simulink model "Task1_Direct_MRAC"  (R2024b)
settings: Solver=ode45  StartTime=0.0  StopTime=60  MaxStep=0.01  RelTol=1e-7  AbsTol=1e-9
Description:
  | Task 1 direct MRAC. The plant, reference model, command, controller, regressor, and adaptive laws are contained in the MATLAB Function block.
  | Set Command Case to 1 for the step command or 2 for the five-tone PE command.
  | Results are shown only in Scope and Display blocks.
settings Model: Creator=LAPTOPASADI  LastModifiedBy=LAPTOPASADI
settings DataIOCC: SaveOutput=off  SignalLogging=off  SaveTime=off  ReturnWorkspaceOutputs=off

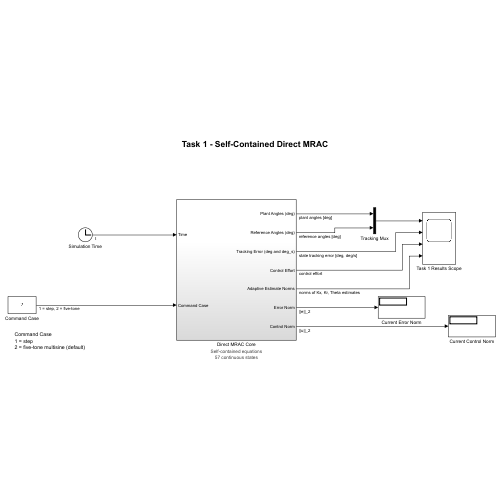
[thumbnail: Simulink's stored preview of the top-level diagram]
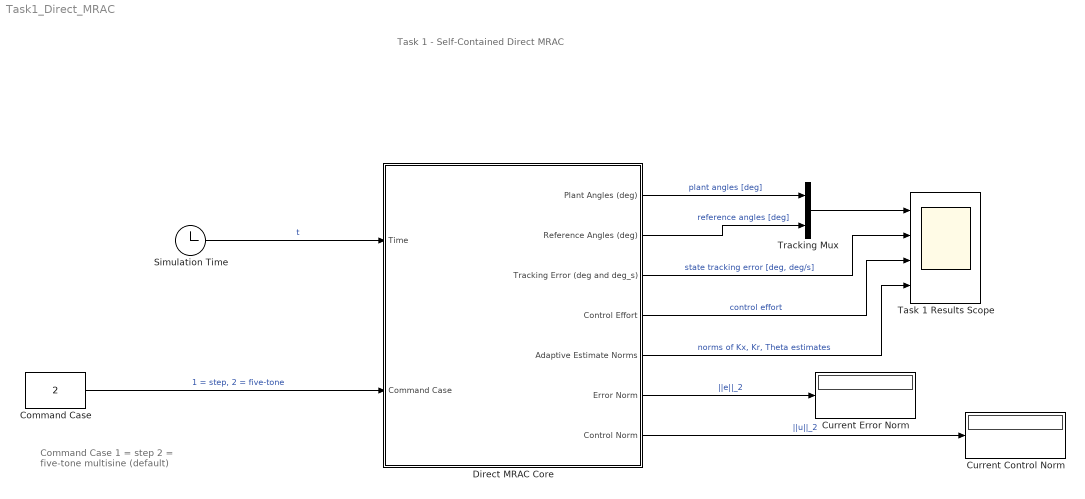
== system Task1_Direct_MRAC ==
  note: Task 1 - Self-Contained Direct MRAC
  note: Command Case
      | 1 = step
      | 2 = five-tone multisine (default)
  Command Case : Constant  Value=2  OutDataTypeStr=double
  Current Control Norm : Display
  Current Error Norm : Display
  Direct MRAC Core : Subsystem
      settings: AttributesFormatString=Self-contained equations\n57 continuous states
  Simulation Time : Clock
  Task 1 Results Scope : Scope  NumInputPorts=4
  Tracking Mux : Mux  Inputs=2
  wires:
  Simulation Time/1 -> Direct MRAC Core/1(Time)  "t"
  Command Case/1 -> Direct MRAC Core/2(Command Case)  "1 = step, 2 = five-tone"
  Direct MRAC Core/1(Plant Angles (deg)) -> Tracking Mux/1  "plant angles [deg]"
  Direct MRAC Core/2(Reference Angles (deg)) -> Tracking Mux/2  "reference angles [deg]"
  Tracking Mux/1 -> Task 1 Results Scope/1
  Direct MRAC Core/3(Tracking Error (deg and deg_s)) -> Task 1 Results Scope/2  "state tracking error [deg, deg/s]"
  Direct MRAC Core/4(Control Effort) -> Task 1 Results Scope/3  "control effort"
  Direct MRAC Core/5(Adaptive Estimate Norms) -> Task 1 Results Scope/4  "norms of Kx, Kr, Theta estimates"
  Direct MRAC Core/6(Error Norm) -> Current Error Norm/1  "||e||_2"
  Direct MRAC Core/7(Control Norm) -> Current Control Norm/1  "||u||_2"

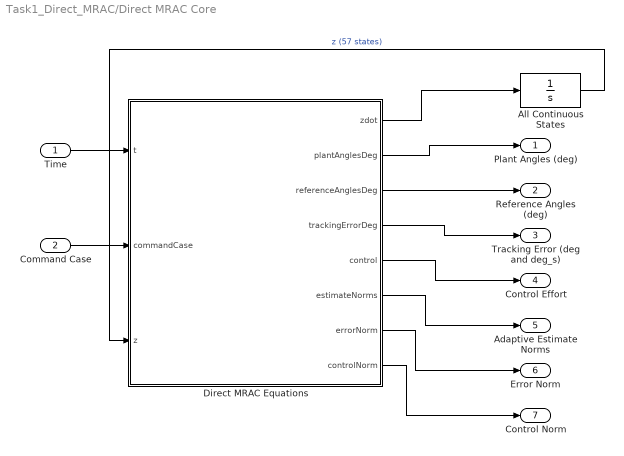
== system Task1_Direct_MRAC/Direct MRAC Core ==
  Time : Inport
  Command Case : Inport  Port=2
  All Continuous States : Integrator  InitialCondition=zeros(57,1)
  Direct MRAC Equations : MATLAB Function  TreatAsAtomicUnit=on
  Plant Angles (deg) : Outport
  Reference Angles (deg) : Outport  Port=2
  Tracking Error (deg and deg_s) : Outport  Port=3
  Control Effort : Outport  Port=4
  Adaptive Estimate Norms : Outport  Port=5
  Error Norm : Outport  Port=6
  Control Norm : Outport  Port=7
  wires:
  Time/1 -> Direct MRAC Equations/1(t)
  Command Case/1 -> Direct MRAC Equations/2(commandCase)
  Direct MRAC Equations/1(zdot) -> All Continuous States/1
  Direct MRAC Equations/2(plantAnglesDeg) -> Plant Angles (deg)/1
  Direct MRAC Equations/6(estimateNorms) -> Adaptive Estimate Norms/1
  Direct MRAC Equations/5(control) -> Control Effort/1
  Direct MRAC Equations/4(trackingErrorDeg) -> Tracking Error (deg and deg_s)/1
  Direct MRAC Equations/3(referenceAnglesDeg) -> Reference Angles (deg)/1
  Direct MRAC Equations/7(errorNorm) -> Error Norm/1
  Direct MRAC Equations/8(controlNorm) -> Control Norm/1
  All Continuous States/1 -> Direct MRAC Equations/3(z)  "z (57 states)"

== matlab function Task1_Direct_MRAC/Direct MRAC Core/Direct MRAC Equations ==
  data: t input; zdot output; commandCase input; z input; plantAnglesDeg output; referenceAnglesDeg output; trackingErrorDeg output; control output; estimateNorms output; errorNorm output; controlNorm output
function [zdot,plantAnglesDeg,referenceAnglesDeg,trackingErrorDeg,control,estimateNorms,errorNorm,controlNorm] = directMRAC(t,commandCase,z)
%#codegen
% Self-contained Task 1 model. No project .m file is called here.

x = z(1:6);
xm = z(7:12);
KxHat = reshape(z(13:30),6,3);
KrHat = reshape(z(31:39),3,3);
ThetaHat = reshape(z(40:57),6,3);

% Step or five-tone command. The command starts at one second.
reference = zeros(3,1);
if t >= 1
    if commandCase < 1.5
        reference = (pi/180)*[5;-5;8];
    else
        tau = t-1;
        weights = [0.30,0.24,0.19,0.15,0.12];
        peaks = (pi/180)*[10;10;15];
        amplitude = peaks*weights;
        frequency = [0.31,0.53,0.79,1.07,1.37; ...
                     0.37,0.61,0.89,1.19,1.43; ...
                     0.43,0.67,0.97,1.27,1.51];
        reference = sum(amplitude.*sin(frequency*tau),2);
    end
end

% Physical plant matrices copied from Main.m.
dOverB = 1.2e-6/3.13e-5;
G = [0,0.175/0.0043,dOverB/0.0043; ...
     0.085/0.0142,0,0; ...
     0,dOverB/0.0176,-0.175/0.0176];
aP = (0.0142-0.0176)/0.0043;
aQ = (0.0176-0.0043)/0.0142;
aR = (0.0043-0.0142)/0.0176;
Htrue = [aP,0,0,-0.01,0,0; ...
         0,aQ,0,0,-0.01,0; ...
         0,0,aR,0,0,-0.01];

p = x(4);
q = x(5);
rBody = x(6);
Phi = [q*rBody;p*rBody;p*q;p;q;rBody];

% Direct MRAC control and nominal plant dynamics.
control = KxHat.'*x + KrHat.'*reference - ThetaHat.'*Phi;
xdot = [x(4:6);G*control+Htrue*Phi];
xmdot = [xm(4:6);-4*xm(1:3)-4*xm(4:6)+4*reference];

% Lyapunov-based adaptive laws.
error = x-xm;
P = [1.125*eye(3),0.125*eye(3); ...
     0.125*eye(3),0.15625*eye(3)];
B = [zeros(3,3);G];
adaptationSignal = error.'*P*B;
KxHatDot = -50*x*adaptationSignal;
KrHatDot = -50*reference*adaptationSignal;
ThetaHatDot = 50*Phi*adaptationSignal;

zdot = [xdot;xmdot;KxHatDot(:);KrHatDot(:);ThetaHatDot(:)];

% Readable outputs for Scope and Display blocks only.
plantAnglesDeg = (180/pi)*x(1:3);
referenceAnglesDeg = (180/pi)*xm(1:3);
trackingErrorDeg = (180/pi)*error;
estimateNorms = [sqrt(sum(KxHat(:).^2)); ...
                 sqrt(sum(KrHat(:).^2)); ...
                 sqrt(sum(ThetaHat(:).^2))];
errorNorm = sqrt(sum(error.^2));
controlNorm = sqrt(sum(control.^2));
end
